simulink model "bloquesT4"  (R2025a)
settings: Solver=ode45  StartTime=0.0  StopTime=10.0  RelTol=1e-3
InitFcn:
  | k = 100
  | m = 10
settings Model: Creator=carlo  LastModifiedBy=carlo

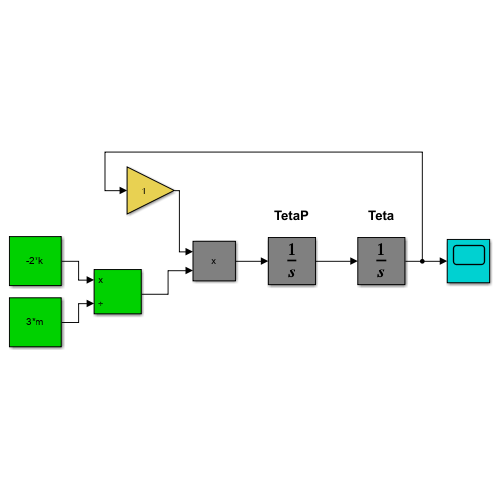
[thumbnail: Simulink's stored preview of the top-level diagram]
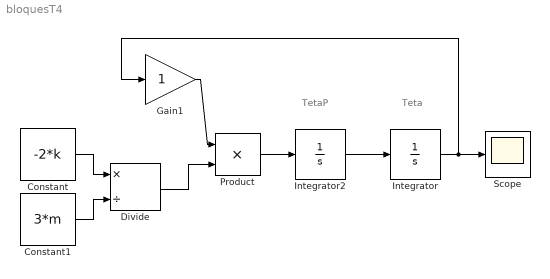
== system bloquesT4 ==
  note: TetaP
  note: Teta
  Constant : Constant  Value=-2*k
  Constant1 : Constant  Value=3*m
  Divide : Product  Inputs=*/
  Gain1 : Gain
  Integrator : Integrator
  Integrator2 : Integrator  InitialCondition=2
  Product : Product
  Scope : Scope
      settings: ActiveDisplayYMinimum=-0.967595483219808  ActiveDisplayYMaximum=0.96805715405171955
  wires:
  Constant/1 -> Divide/1
  Constant1/1 -> Divide/2
  Integrator2/1 -> Integrator/1
  Integrator/1 -> Gain1/1, Scope/1
  Divide/1 -> Product/2
  Gain1/1 -> Product/1
  Product/1 -> Integrator2/1
